simulink model "lidar_webcam_obfind"  (Simulink 7.3)
settings: Solver=FixedStepDiscrete  StartTime=0.0  StopTime=inf  MaxStep=0.2  RelTol=1e-3
libraries: vipstatistics x1, simulink x1
settings Model: Creator=gclayton  LastModifiedBy=wildcat
settings DebuggingCC: InheritedTsInSrcMsg=none
settings RTWCC: SystemTargetFile=rlnx.tlc  GenCodeOnly=on  TemplateMakefile=rlnx_ubuntu.tmf  Description=Linux Real-Time Target  ProcessScript=rlnx_make_rtw_hook
settings RTWCC: CustomInclude=|
  | /usr/local/include/opencv/
  | /usr/local/include/
settings CodeAppCC: GenerateComments=off  SimulinkBlockComments=off
settings STFCustomTargetCC: ModelReferenceCompliant=off  MatFileLogging=on  SystemTargetFile=rlnx.tlc
settings GRTTargetCC: ModelReferenceCompliant=off  ParMdlRefBuildCompliant=off  CompOptLevelCompliant=off
settings CustomProperty: DataType=string  Value=-lm -ldl /usr/local/lib/libopencv_highgui.so.2.4 /usr/local/lib/libopencv_core.so.2.4 /usr/local/lib/libopencv_imgproc.so.2.4 -lc_urg -lc_urg_connection -lc_urg_system -lphidget21
settings EnumStrPairs: String=PC

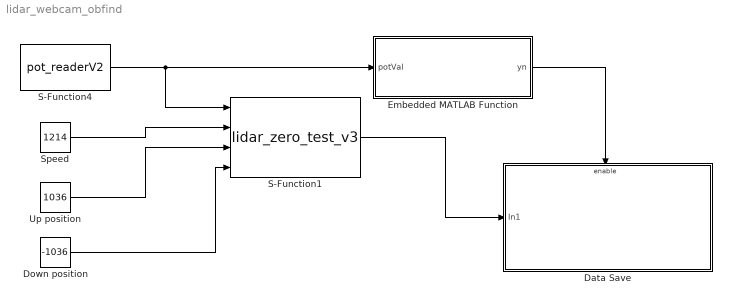
== system lidar_webcam_obfind ==
  Data Save : Subsystem  TreatAsAtomicUnit=on
  Down position : Constant  Value=-1036  OutDataType=fixdt(1, 16)  OutScaling=2^0
  Embedded MATLAB Function : Stateflow chart
  S-Function1 : S-Function  FunctionName=lidar_zero_test_v3  EnableBusSupport=off
  S-Function4 : S-Function  FunctionName=pot_readerV2  EnableBusSupport=off
  Speed : Constant  Value=1214  OutDataType=fixdt(1, 16)  OutScaling=2^0
  Up position : Constant  Value=1036  OutDataType=fixdt(1, 16)  OutScaling=2^0
  wires:
  Speed/1 -> S-Function1/2
  Up position/1 -> S-Function1/3
  Down position/1 -> S-Function1/4
  S-Function4/1 -> S-Function1/1, Embedded MATLAB Function/1(potVal)
  S-Function1/1 -> Data Save/1(In1)
  Embedded MATLAB Function/1(yn) -> Data Save/Enable

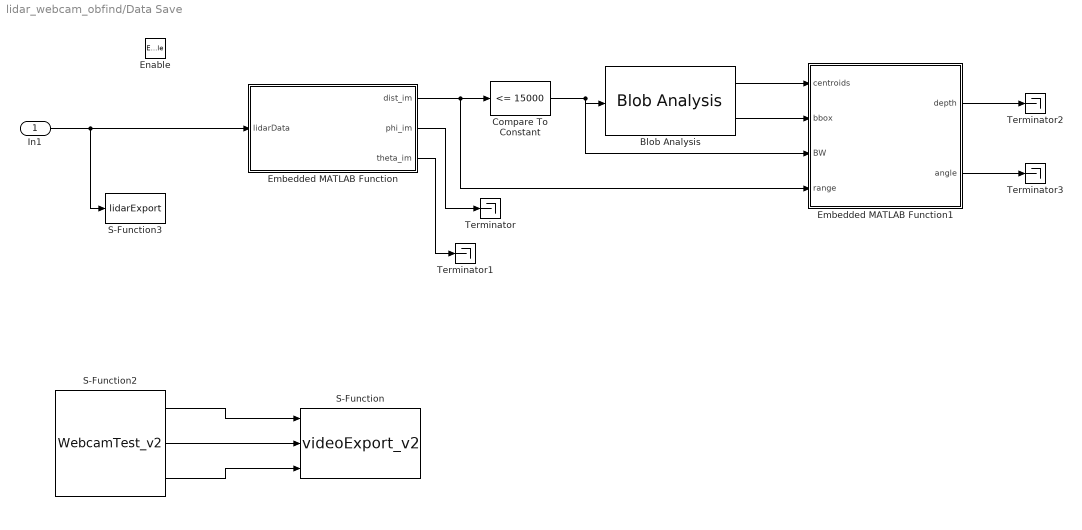
== system lidar_webcam_obfind/Data Save ==
  In1 : Inport  OutDataType=fixdt(1, 16)  OutScaling=2^0
  Enable : EnablePort
  Blob Analysis : vipstatistics/Blob Analysis  DialogController=vipDDGCreate  DialogControllerArgs=DataTag0  area=off  centroid=on  bBox=on  majorAxis=off  minorAxis=off  angle=off  eccentricity=off  equivDiameterSq=off  extent=off  perimeter=off  maxBlobs=50  warnIfNumBlobsExceeded=on  isCount=off  useMinArea=on  minArea=30  useMaxArea=off  maxArea=intmax('uint32')  excludeBorderBlob=on  outDT=double  isOutVarDim=off  isFill=on  fillValues=-1  conn=8  isLabel=off  outputMode=Binary point scaling  outputWordLength=32  outputFracLength=16  firstCoeffMode=Binary point scaling  firstCoeffWordLength=16  firstCoeffFracLength=14  secondCoeffMode=Binary point scaling  secondCoeffWordLength=32  secondCoeffFracLength=16  accumMode=Binary point scaling  accumWordLength=32  accumFracLength=0  prodOutputMode=Binary point scaling  prodOutputWordLength=32  prodOutputFracLength=16  roundingMode=Floor  overflowMode=off
  Compare To Constant : simulink/Logic and Bit Operations/Compare To Constant  SystemSampleTime=-1  relop=<=  const=15000  LogicOutDataTypeMode=boolean  ZeroCross=off
  Embedded MATLAB Function : Stateflow chart
  Embedded MATLAB Function1 : Stateflow chart
  S-Function : S-Function  FunctionName=videoExport_v2  EnableBusSupport=off
  S-Function2 : S-Function  FunctionName=WebcamTest_v2  EnableBusSupport=off
  S-Function3 : S-Function  FunctionName=lidarExport  EnableBusSupport=off
  Terminator{,1..3} (4 alike) : Terminator
  wires:
  S-Function2/3 -> S-Function/3
  S-Function2/2 -> S-Function/2
  S-Function2/1 -> S-Function/1
  In1/1 -> Embedded MATLAB Function/1(lidarData), S-Function3/1
  Embedded MATLAB Function/1(dist_im) -> Compare To Constant/1, Embedded MATLAB Function1/4(range)
  Embedded MATLAB Function/2(phi_im) -> Terminator/1
  Embedded MATLAB Function/3(theta_im) -> Terminator1/1
  Compare To Constant/1 -> Blob Analysis/1, Embedded MATLAB Function1/3(BW)
  Blob Analysis/1 -> Embedded MATLAB Function1/1(centroids)
  Blob Analysis/2 -> Embedded MATLAB Function1/2(bbox)
  Embedded MATLAB Function1/2(angle) -> Terminator3/1
  Embedded MATLAB Function1/1(depth) -> Terminator2/1

== matlab function Data Save/Embedded MATLAB Function ==
  data: lidarData input double; dist_im output double; phi_im output double; theta_im output double
function [dist_im, phi_im, theta_im] = image_creator(lidarData)
%#eml

% Define variables based on gimbal system and scan pattern
ScanNum = 65;
DataLength = 1080*ScanNum;
h = 36.3;

% Define Data sizes
phim = zeros(1,DataLength);
thetam = zeros(1,DataLength);
distm = zeros(1,DataLength);
dist_im = zeros(ScanNum,600);
phi_im = zeros(ScanNum,600);
theta_im = zeros(ScanNum,600);


%Define phi_rad: angles corresponding to one lidar scan
l = 1:1080;
phi_rad = (-45 + 0.25*l)*pi/180;

% Repeat phim for number of scans
for i = 1:ScanNum
        
    for j = 1 : 1080
        phi_val = 1080*(i-1) + j;
        phim(1,phi_val) = phi_rad(1,j);
    end
end

% Theta changes from -45 to 45 degrees over the duration of the scan
theta_min = -45*pi/180;
theta_max = 45*pi/180;
theta_step = (theta_max - theta_min)/DataLength;
thetam = [theta_max : -theta_step : (theta_min+theta_step)];

% Distance matrix is directly from lidar data
distm = lidarData';


% Create images for distance, phi, and theta
for i2 = 1:ScanNum
    for j2 = 1:600
        dist_im(i2,j2) = distm(1, 240+j2 + 1080*(i2-1));
        phi_im(i2,j2) = phim(1, 240+j2 + 1080*(i2-1));
        theta_im(i2,j2) = thetam(1, 240+j2 + 1080*(i2-1));
    end
    
end

== matlab function Embedded MATLAB Function ==
  data: potVal input double; yn output double
function yn = check_pot_val(potVal)
%#eml

% Pot value may initially be zero.
% Check for this and output a 1 or zero to 
% control whether the rest of model runs
if (potVal == 0)
    yn = 0;
else
    yn = 1;
end

== matlab function Data Save/Embedded MATLAB Function1 ==
  data: centroids input double; depth output double; bbox input double; BW input double; range input double; angle output double
function [depth, angle]  = depth_and_range(centroids, bbox, BW, range)
%Written by Anderson Lebbad on June 25, 2014
%Last Edited:

%This function creates a histogram of the color region of a detected object
%identified in a binary image within a bounding box

%Initialize variables
[M,N] = size(bbox);
RunAve = zeros(M,1);
%Needs to be updated for raster angles
FieldOfView = 62*pi/180;
wFrame = 640;
angle = (centroids(:,1)-wFrame/2)*FieldOfView/wFrame;

%Loop for multiple identified objects
for k=1:M
    pixels = 0;
    
    %Parse bbox data
    left = bbox(k,1);
    right = left + bbox(k,3) - 1;
    bottom = bbox(k,2);
    top = bottom + bbox(k,4) - 1;
    
    %Check to see if valid bbox is found
    if left~=-1
        %Scan the detected region of the binary image and generate histograms
        for j=left:right
            for i=bottom:top
                if BW(i,j) == 1
                    pixels = pixels + 1;
                    RunAve(k) = ((pixels-1)/pixels)*RunAve(k) + (1/pixels)*double(range(i,j));
                end
            end
        end
    end
end

%Means must be integers to use in Bayes Filter
depth = uint8(RunAve);

end
